simulink model "bldc_model_bst"  (R2014b)
settings: Solver=ode3  StartTime=0.0  StopTime=120  FixedStep=0.01  RelTol=1e-3
undefined symbols (not defined in the file): rpm2rps, rps2rpm
libraries: simulink x1
settings Model: Creator=root  LastModifiedBy=root

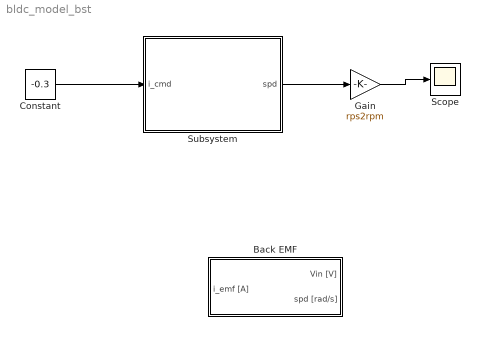
== system bldc_model_bst ==
  Back EMF : Subsystem  TreatAsAtomicUnit=on
  Constant : Constant  Value=-0.3
  Gain : Gain  Gain=rps2rpm
  Scope : Scope
  Subsystem : Subsystem  mask{Ke=0.002115/(1*(2*pi/60)), Km=0.02020, R=2.5, f_abc=[1.58979E-11, 2.06636E-7, 5.69935E-4], J=0.0009785480, spd_0=5000*rpm2rps, i_max=0.9, V_in=23.0}
      mask prompts: Ke "Back-EMF Constant [V/(rad/s)]"; Km "Motor Torque Constant [Nm/A]"; R "Motor Resistance [Ohm]"; f_abc "Friction Coefficients"; J "Moment of Inertia [kgm2]"; spd_0 "Initial Speed [rad/s]"; i_max "Maximum Current [A]"; V_in "Input Voltage [V]"
  wires:
  Constant/1 -> Subsystem/1(i_cmd)
  Subsystem/1(spd) -> Gain/1
  Gain/1 -> Scope/1

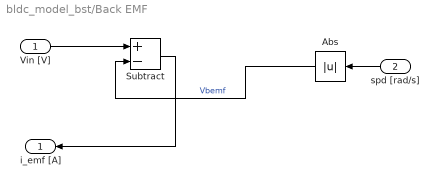
== system bldc_model_bst/Back EMF ==
  Vin [V] : Inport
  spd [rad/s] : Inport  Port=2
  Abs : Abs
  Subtract : Sum  Inputs=+-
  i_emf [A] : Outport
  wires:
  Vin [V]/1 -> Subtract/1
  Subtract/1 -> i_emf [A]/1
  spd [rad/s]/1 -> Abs/1
  Abs/1 -> Subtract/2  "Vbemf"

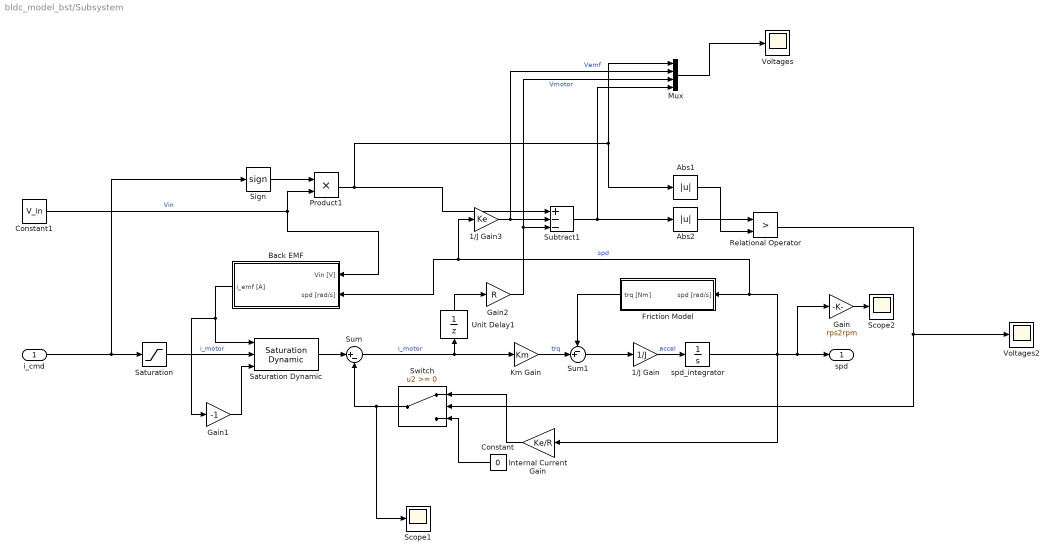
== system bldc_model_bst/Subsystem ==
  i_cmd : Inport
  1/J Gain : Gain  Gain=1/J
  1/J Gain3 : Gain  Gain=Ke
  Abs1 : Abs
  Abs2 : Abs
  Back EMF : Subsystem
  Constant : Constant  Value=0
  Constant1 : Constant  Value=V_in
  Friction Model : Subsystem
  Gain : Gain  Gain=rps2rpm
  Gain1 : Gain  Gain=-1
  Gain2 : Gain  Gain=R
  Internal Current Gain : Gain  Gain=Ke/R
  Km Gain : Gain  Gain=Km
  Mux : Mux
  Product1 : Product
  Relational Operator : RelationalOperator  Operator=>  OutDataTypeStr=boolean
  Saturation : Saturate  UpperLimit=i_max  LowerLimit=-i_max
  Saturation Dynamic : simulink/Discontinuities/Saturation Dynamic  OutMin=[]  OutMax=[]  OutDataTypeStr=Inherit: Same as second input  OutDataType=fixdt(1, 16)  OutScaling=2^-10  DoSatur=off
  Scope1 : Scope
      settings: TimeRange=12.402  YMin=-1.5  YMax=-0.8999999999999999
  Scope2 : Scope
      settings: SaveName=ScopeData3
  Sign : Signum
  Subtract1 : Sum  Inputs=+--
  Sum : Sum  Inputs=|+-
  Sum1 : Sum  Inputs=-+|
  Switch : Switch
  Unit Delay1 : UnitDelay  SampleTime=-1
  Voltages : Scope
      settings: ShowLegends=on  TimeRange=30  YMin=-25  YMax=0  SaveName=ScopeData4  ScrollMode=on
  Voltages2 : Scope
      settings: ShowLegends=on  TimeRange=30  YMin=-10  YMax=15  SaveName=ScopeData5  ScrollMode=on
  spd_integrator : Integrator  InitialCondition=spd_0
  spd : Outport
  wires:
  Km Gain/1 -> Sum1/2  "trq"
  spd_integrator/1 -> Internal Current Gain/1, spd/1, Gain/1, Friction Model/1(spd [rad/s]), 1/J Gain3/1, Back EMF/2(spd [rad/s])  "spd"
  Sum1/1 -> 1/J Gain/1
  Switch/1 -> Sum/2, Scope1/1
  Sum/1 -> Km Gain/1, Unit Delay1/1  "i_motor"
  i_cmd/1 -> Sign/1, Saturation/1
  Internal Current Gain/1 -> Switch/1
  1/J Gain/1 -> spd_integrator/1  "accel"
  Constant1/1 -> Product1/2, Back EMF/1(Vin [V])  "Vin"
  Gain/1 -> Scope2/1
  Saturation/1 -> Saturation Dynamic/2  "i_motor"
  Saturation Dynamic/1 -> Sum/1
  Gain1/1 -> Saturation Dynamic/3
  Friction Model/1(trq [Nm]) -> Sum1/1
  Gain2/1 -> Mux/3, Subtract1/3  "Vmotor"
  Mux/1 -> Voltages/1
  Subtract1/1 -> Mux/4, Abs2/1
  1/J Gain3/1 -> Mux/2, Subtract1/2  "Vemf"
  Constant/1 -> Switch/3
  Relational Operator/1 -> Voltages2/1, Switch/2
  Sign/1 -> Product1/1
  Product1/1 -> Abs1/1, Mux/1, Subtract1/1
  Abs1/1 -> Relational Operator/2
  Abs2/1 -> Relational Operator/1
  Unit Delay1/1 -> Gain2/1
  Back EMF/1(i_emf [A]) -> Saturation Dynamic/1, Gain1/1

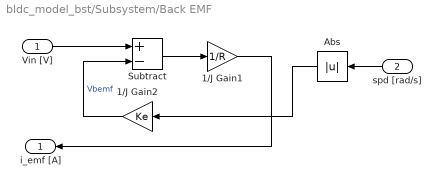
== system bldc_model_bst/Subsystem/Back EMF ==
  Vin [V] : Inport
  spd [rad/s] : Inport  Port=2
  1/J Gain1 : Gain  Gain=1/R
  1/J Gain2 : Gain  Gain=Ke
  Abs : Abs
  Subtract : Sum  Inputs=+-
  i_emf [A] : Outport
  wires:
  Vin [V]/1 -> Subtract/1
  1/J Gain1/1 -> i_emf [A]/1
  Subtract/1 -> 1/J Gain1/1
  spd [rad/s]/1 -> Abs/1
  1/J Gain2/1 -> Subtract/2  "Vbemf"
  Abs/1 -> 1/J Gain2/1

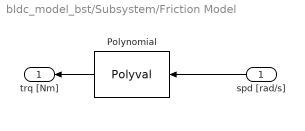
== system bldc_model_bst/Subsystem/Friction Model ==
  spd [rad/s] : Inport
  Polynomial : Polyval  Coefs=f_abc
  trq [Nm] : Outport
  wires:
  spd [rad/s]/1 -> Polynomial/1
  Polynomial/1 -> trq [Nm]/1
